simulink model "sensor_fusion"  (R2017b)
settings: Solver=ode45  StartTime=0.0  StopTime=inf  FixedStep=0.1  RelTol=1e-3  EnableMultiTasking=on
PreLoadFcn:
  | RTWConfigurationCB('preloadfcn', bdroot);
InitFcn:
  | parameterVehicle
  | parameterGNC
StopFcn:
  | %myAnimation(xActEst,yActEst,thetaActEst,X_array,Y_array,rp1,rp2)
  | myStopFcn2sim(xEst,yEst,X_array,Y_array,rp1,rp2)
values from neighbouring files (symbols this model uses):
  bDR = 1*b    [parameterGNC.m]
  dcArrayC = [-240 -220 -200 -150 -100 -80 -60 -50 -40 0 40 50    60    80   100   150 200 220 240]    [parameterGNC.m]
  eTickDR = eTick    [parameterGNC.m]
  KP1 = 15    [parameterGNC.m]
  KP2 = 100    [parameterGNC.m]
  rNominalDR = rNominal    [parameterGNC.m]
  rp1 = 0.5    [parameterGNC.m]
  rp2 = 0.2    [parameterGNC.m]
  Tau1 = 0.01    [parameterGNC.m]
  Tau2 = 0.1    [parameterGNC.m]
  TauEncoderDR = 0.01    [parameterGNC.m]
  Tsample = 1/100    (= 0.01)    [parameterGNC.m]
  TsampleEncoderDR = TsampleEncoder    [parameterGNC.m]
  Vcom = 3*VmaxDR/4    [parameterGNC.m]
  wArrayC = [-4.6279   -4.1707   -3.6703   -2.4511   -1.0693   -0.8382   -0.4348   -0.3287 -0.000001 0 0.000001 0.3292    0.4343    0.8065    1.0897    2.3927    3.6855    4.2037    4.6126]./rNominal    [parameterGNC.m]
  X_array = [1 1 0 0]    [parameterGNC.m]
  Y_array = [0 1 1 0]    [parameterGNC.m]
undefined symbols (not defined in the file or in its folder): DiscIntNeverNeededParam
libraries: simulink x17, robotlib x10, aerolibanimutils x1
CloseFcn:
  | rtwprivate ssgencode ModelCloseRequest track_vehicle6_v2
settings Model: Creator=Dogan  LastModifiedBy=uvs4
settings DataIOCC: LimitDataPoints=on  SaveFormat=Array  SignalLoggingSaveFormat=ModelDataLogs
settings OptimizationCC: ExpressionDepthLimit=2147483647  InitFltsAndDblsToZero=on  LifeSpan=inf
settings DebuggingCC: SaveWithParameterizedLinksMsg=none  UnderspecifiedInitializationDetection=Classic  MergeDetectMultiDrivingBlocksExec=none  SignalResolutionControl=TryResolveAllWithWarning  SolverPrmCheckMsg=warning  MultiTaskDSMMsg=warning  MultiTaskCondExecSysMsg=none  FcnCallInpInsideContextMsg=warning  StateNameClashWarn=warning  SFUnexpectedBacktrackingDiag=warning  SFNoUnconditionalDefaultTransitionDiag=warning  SFExecutionAtInitializationDiag=none
settings HardwareCC: ProdBitPerLong=64  ProdLargestAtomicFloat=None  ProdHWDeviceType=Intel->x86-64  TargetHWDeviceType=32-bit Generic
settings ModelReferenceCC: PropagateSignalLabelsOutOfModel=off
settings SFSimCC: SimParseCustomCode=off
settings RTWCC: Description=Generic Real-Time Target
settings CodeAppCC: GenerateComments=off  SimulinkBlockComments=off
settings GRTTargetCC: TargetLangStandard=C89/C90 (ANSI)  GeneratePreprocessorConditionals=Disable all
settings ConfigComp: CovMetricSettings=dw  CovHtmlReporting=on  CovSaveCumulativeToWorkspaceVar=on  CovSaveSingleToWorkspaceVar=on  CovExternalEMLEnable=off

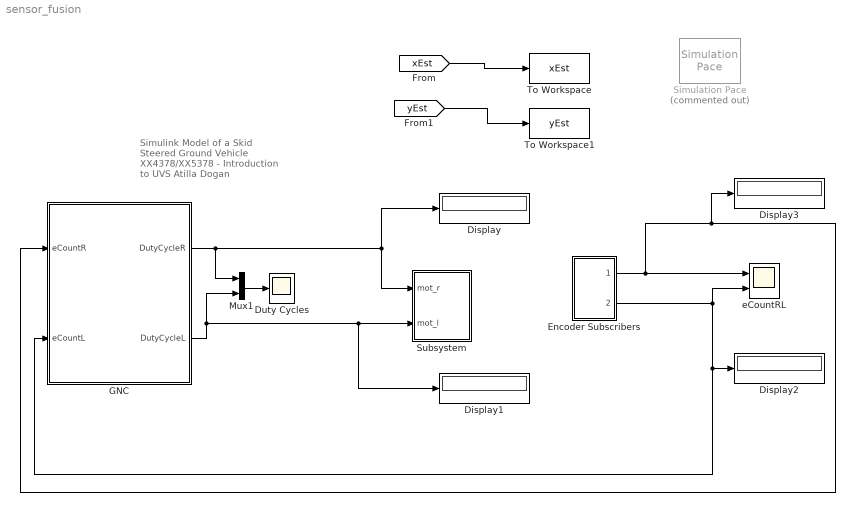
== system sensor_fusion ==
  note: Simulink Model of a Skid Steered Ground Vehicle
      | XX4378/XX5378 - Introduction to UVS
      | Atilla Dogan
  Display{,1..3} (4 alike) : Display
  Duty Cycles : Scope
  Encoder Subscribers : Subsystem
  GNC : Subsystem
  Mux1 : Mux  Inputs=2
  Simulation Pace : aerolibanimutils/Simulation Pace  Commented=on  SimulationPace=1  SleepMode=MATLAB Thread  OutputPaceError=off  SampleTime=1/30
  Subsystem : Subsystem
  To Workspace : ToWorkspace  VariableName=xEst  SaveFormat=Structure With Time  SampleTime=-1
  To Workspace1 : ToWorkspace  VariableName=yEst  SaveFormat=Structure With Time  SampleTime=-1
  eCountRL : Scope  NumInputPorts=2
  wires:
  Mux1/1 -> Duty Cycles/1
  [xEst] -> To Workspace/1
  [yEst] -> To Workspace1/1
  GNC/1(DutyCycleR) -> Mux1/1, Display/1, Subsystem/1(mot_r)
  GNC/2(DutyCycleL) -> Subsystem/2(mot_l), Display1/1, Mux1/2
  Encoder Subscribers/1(enco_R) -> Display3/1, GNC/1(eCountR), eCountRL/1
  Encoder Subscribers/2(enco_L) -> Display2/1, GNC/2(eCountL), eCountRL/2

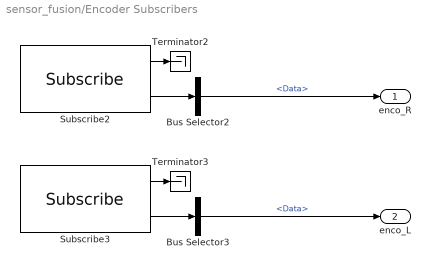
== system sensor_fusion/Encoder Subscribers ==
  Bus Selector2 : BusSelector  OutputSignals=Data
  Bus Selector3 : BusSelector  OutputSignals=Data
  Subscribe2 : robotlib/Subscribe  SourceLibraryInfo=This block requires Robotics System Toolbox  topicSource=Specify your own  topic=/enco_R  messageType=std_msgs/Int16  sampleTime=-1  messageQueueLength=1
      settings: SourceProductBaseCode=RO
  Subscribe3 : robotlib/Subscribe  SourceLibraryInfo=This block requires Robotics System Toolbox  topicSource=Specify your own  topic=/enco_L  messageType=std_msgs/Int16  sampleTime=-1  messageQueueLength=1
      settings: SourceProductBaseCode=RO
  Terminator2 : Terminator
  Terminator3 : Terminator
  enco_R : Outport
  enco_L : Outport  Port=2
  wires:
  Subscribe2/2 -> Bus Selector2/1
  Subscribe2/1 -> Terminator2/1
  Subscribe3/2 -> Bus Selector3/1
  Bus Selector3/1 -> enco_L/1  "<Data>"
  Bus Selector2/1 -> enco_R/1  "<Data>"
  Subscribe3/1 -> Terminator3/1

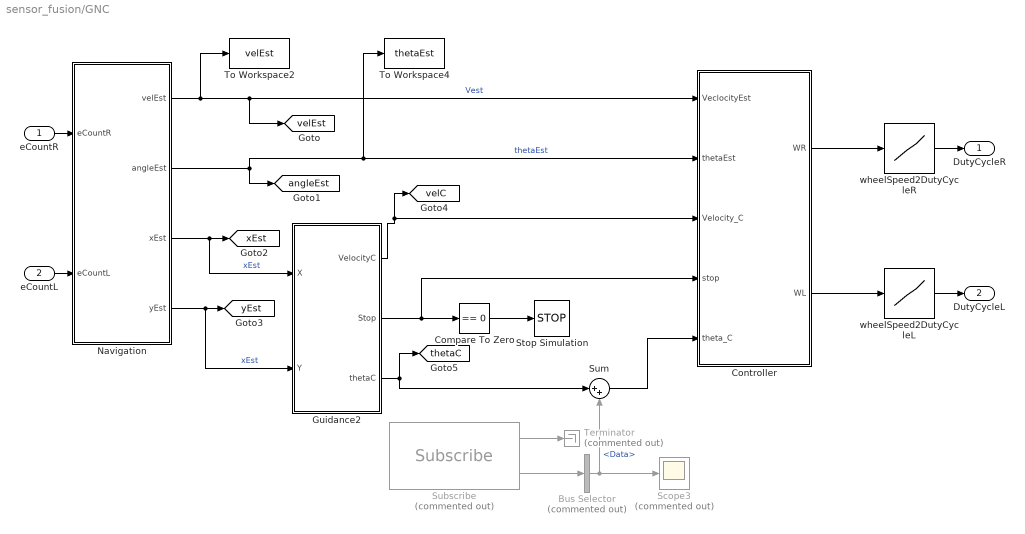
== system sensor_fusion/GNC ==
  eCountR : Inport
  eCountL : Inport  Port=2
  Bus Selector : BusSelector  Commented=on  OutputSignals=Data
  Compare To Zero : simulink/Logic and Bit Operations/Compare To Zero  relop===  OutDataTypeStr=boolean
  Controller : Subsystem
  Guidance2 : Subsystem
  "Navigation " : Subsystem
  Scope3 : Scope  Commented=on
  Stop Simulation : Stop
  Subscribe : robotlib/Subscribe  Commented=on  SourceLibraryInfo=This block requires Robotics System Toolbox  topicSource=Specify your own  topic=/theta_deflection  messageType=std_msgs/Float64  sampleTime=-1  messageQueueLength=1
      settings: SourceProductBaseCode=RO
  Sum : Sum  Inputs=|++
  Terminator : Terminator  Commented=on
  To Workspace2 : ToWorkspace  VariableName=velEst  SampleTime=-1
      settings: Save2DSignal=2-D array (concatenate along first dimension)
  To Workspace4 : ToWorkspace  VariableName=thetaEst  SampleTime=-1
      settings: Save2DSignal=2-D array (concatenate along first dimension)
  wheelSpeed2DutyCycleL : Lookup  InputValues=wArrayC  Table=dcArrayC  LookUpMeth=Interpolation-Use End Values
  wheelSpeed2DutyCycleR : Lookup  InputValues=wArrayC  Table=dcArrayC  LookUpMeth=Interpolation-Use End Values
  DutyCycleR : Outport
  DutyCycleL : Outport  Port=2
  tag scope: angleEst=global, thetaC=global, velC=global, velEst=global, xEst=global, yEst=global
  wires:
  Guidance2/2(Stop) -> Controller/4(stop), Compare To Zero/1
  Controller/1(WR) -> wheelSpeed2DutyCycleR/1
  "Navigation "/4(yEst) -> Guidance2/2(Y), [yEst]  "xEst"
  "Navigation "/3(xEst) -> Guidance2/1(X), [xEst]  "xEst"
  "Navigation "/2(angleEst) -> To Workspace4/1, Controller/2(thetaEst), [angleEst]  "thetaEst"
  "Navigation "/1(velEst) -> To Workspace2/1, Controller/1(VeclocityEst), [velEst]  "Vest"
  eCountL/1 -> "Navigation "/2(eCountL)
  eCountR/1 -> "Navigation "/1(eCountR)
  Guidance2/1(VelocityC) -> Controller/3(Velocity_C), [velC]
  wheelSpeed2DutyCycleR/1 -> DutyCycleR/1
  Controller/2(WL) -> wheelSpeed2DutyCycleL/1
  wheelSpeed2DutyCycleL/1 -> DutyCycleL/1
  Compare To Zero/1 -> Stop Simulation/1
  Guidance2/3(thetaC) -> Sum/1, [thetaC]
  Subscribe/1 -> Terminator/1
  Subscribe/2 -> Bus Selector/1
  Bus Selector/1 -> Sum/2, Scope3/1  "<Data>"
  Sum/1 -> Controller/5(theta_C)

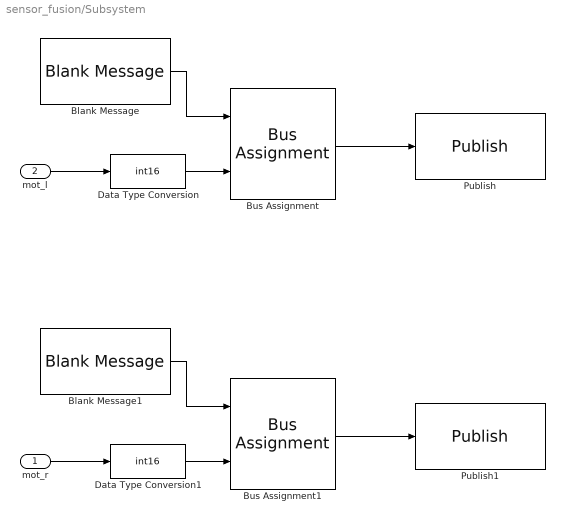
== system sensor_fusion/Subsystem ==
  mot_r : Inport
  mot_l : Inport  Port=2
  Blank Message : robotlib/Blank Message  SourceLibraryInfo=This block requires Robotics System Toolbox  messageType=std_msgs/Int16  SampleTime=inf
      settings: SourceProductBaseCode=RO
  Blank Message1 : robotlib/Blank Message  SourceLibraryInfo=This block requires Robotics System Toolbox  messageType=std_msgs/Int16  SampleTime=inf
      settings: SourceProductBaseCode=RO
  Bus Assignment : BusAssignment  AssignedSignals=Data
  Bus Assignment1 : BusAssignment  AssignedSignals=Data
  Data Type Conversion : DataTypeConversion  OutDataTypeStr=int16
  Data Type Conversion1 : DataTypeConversion  OutDataTypeStr=int16
  Publish : robotlib/Publish  SourceLibraryInfo=This block requires Robotics System Toolbox  topicSource=Specify your own  topic=/pwm_cmd_l  messageType=std_msgs/Int16  messageQueueLength=1
      settings: SourceProductBaseCode=RO
  Publish1 : robotlib/Publish  SourceLibraryInfo=This block requires Robotics System Toolbox  topicSource=Specify your own  topic=/pwm_cmd_r  messageType=std_msgs/Int16  messageQueueLength=1
      settings: SourceProductBaseCode=RO
  wires:
  Bus Assignment/1 -> Publish/1
  Data Type Conversion/1 -> Bus Assignment/2
  Blank Message/1 -> Bus Assignment/1
  mot_l/1 -> Data Type Conversion/1
  mot_r/1 -> Data Type Conversion1/1
  Blank Message1/1 -> Bus Assignment1/1
  Data Type Conversion1/1 -> Bus Assignment1/2
  Bus Assignment1/1 -> Publish1/1

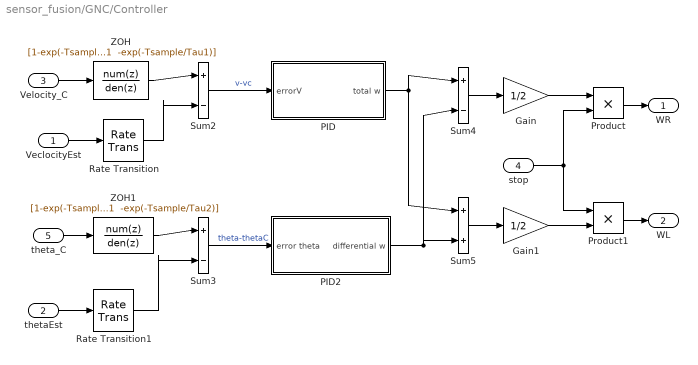
== system sensor_fusion/GNC/Controller ==
  VeclocityEst : Inport
  thetaEst : Inport  Port=2
  Velocity_C : Inport  Port=3
  stop : Inport  Port=4
  theta_C : Inport  Port=5
  Gain : Gain  Gain=1/2
  Gain1 : Gain  Gain=1/2
  PID : Subsystem
  PID2 : Subsystem
  Product : Product  RndMeth=Zero
  Product1 : Product  RndMeth=Zero
  Rate Transition : RateTransition  Deterministic=off
  Rate Transition1 : RateTransition  Deterministic=off
  Sum2 : Sum  Inputs=|+|-|  SampleTime=Tsample
  Sum3 : Sum  Inputs=|+|-|  SampleTime=Tsample
  Sum4 : Sum  Inputs=+|-
  Sum5 : Sum  Inputs=+|+
  ZOH : DiscreteTransferFcn  Numerator=[1-exp(-Tsample/Tau1)]  Denominator="[1  -exp(-Tsample/Tau1)]"  SampleTime=Tsample
  ZOH1 : DiscreteTransferFcn  Numerator=[1-exp(-Tsample/Tau2)]  Denominator="[1  -exp(-Tsample/Tau2)]"  SampleTime=Tsample
  WR : Outport
  WL : Outport  Port=2
  wires:
  Product1/1 -> WL/1
  Product/1 -> WR/1
  Sum5/1 -> Gain1/1
  stop/1 -> Product/2, Product1/1
  Sum4/1 -> Gain/1
  PID2/1(differential w) -> Sum5/2, Sum4/2
  PID/1(total w) -> Sum5/1, Sum4/1
  theta_C/1 -> ZOH1/1
  thetaEst/1 -> Rate Transition1/1
  Velocity_C/1 -> ZOH/1
  VeclocityEst/1 -> Rate Transition/1
  Sum2/1 -> PID/1(errorV)  "v-vc"
  Sum3/1 -> PID2/1(error theta)  "theta-thetaC"
  ZOH/1 -> Sum2/1
  Rate Transition/1 -> Sum2/2
  ZOH1/1 -> Sum3/1
  Rate Transition1/1 -> Sum3/2
  Gain/1 -> Product/1
  Gain1/1 -> Product1/2

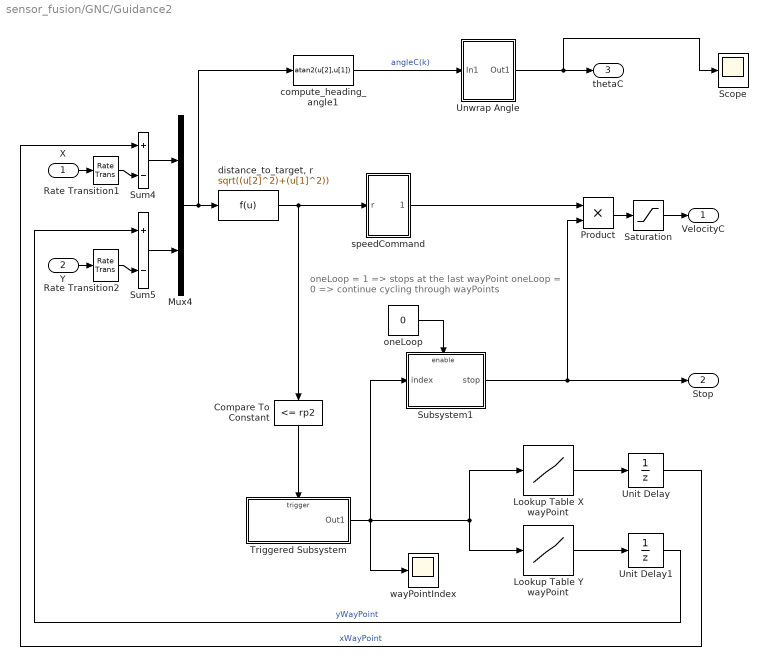
== system sensor_fusion/GNC/Guidance2 ==
  note: oneLoop = 1 => stops at the last wayPoint
      | oneLoop = 0 => continue cycling through wayPoints
  X : Inport
  Y : Inport  Port=2
  Compare To Constant : simulink/Logic and Bit Operations/Compare To Constant  relop=<=  const=rp2  OutDataTypeStr=uint8  ZeroCross=off
  Lookup Table X wayPoint : Lookup  InputValues=[1:length(X_array)]  Table=X_array  LookUpMeth=Interpolation-Use End Values  OutDataTypeStr=double
  Lookup Table Y wayPoint : Lookup  InputValues=[1:length(Y_array)]  Table=Y_array  LookUpMeth=Interpolation-Use End Values  OutDataTypeStr=double
  Mux4 : Mux  Inputs=2
  Product : Product  RndMeth=Zero
  Rate Transition1 : RateTransition
  Rate Transition2 : RateTransition
  Saturation : Saturate  UpperLimit=Vcom  LowerLimit=0  SampleTime=Tsample
  Scope : Scope
  Subsystem1 : Subsystem
  Sum4 : Sum  Inputs=|+|-|
  Sum5 : Sum  Inputs=|+|-|
  Triggered Subsystem : Subsystem  TreatAsAtomicUnit=on
  Unit Delay : UnitDelay  SampleTime=Tsample
  Unit Delay1 : UnitDelay  SampleTime=Tsample
  Unwrap Angle : Subsystem
  compute_heading_angle1 : Fcn  Expr=atan2(u[2],u[1])  SampleTime=Tsample
  "distance_to_target, r" : Fcn  Expr=sqrt((u[2]^2)+(u[1]^2))  SampleTime=Tsample
  oneLoop : Constant  Value=0  OutDataTypeStr=uint32  SampleTime=Tsample
  speedCommand : Subsystem
  wayPointIndex : Scope
  VelocityC : Outport
  Stop : Outport  Port=2
  thetaC : Outport  Port=3
  wires:
  speedCommand/1(Vdes) -> Product/1
  Sum4/1 -> Mux4/1
  "distance_to_target, r"/1 -> Compare To Constant/1, speedCommand/1(r)
  Lookup Table X wayPoint/1 -> Unit Delay/1
  Lookup Table Y wayPoint/1 -> Unit Delay1/1
  X/1 -> Rate Transition1/1
  Y/1 -> Rate Transition2/1
  Sum5/1 -> Mux4/2
  Compare To Constant/1 -> Triggered Subsystem/Trigger
  Triggered Subsystem/1(Out1) -> Subsystem1/1(index), wayPointIndex/1, Lookup Table X wayPoint/1, Lookup Table Y wayPoint/1
  Unit Delay/1 -> Sum4/1  "xWayPoint"
  Unit Delay1/1 -> Sum5/1  "yWayPoint"
  Saturation/1 -> VelocityC/1
  Rate Transition1/1 -> Sum4/2
  Rate Transition2/1 -> Sum5/2
  Product/1 -> Saturation/1
  Subsystem1/1(stop) -> Product/2, Stop/1
  oneLoop/1 -> Subsystem1/Enable
  Mux4/1 -> compute_heading_angle1/1, "distance_to_target, r"/1
  compute_heading_angle1/1 -> Unwrap Angle/1(In1)  "angleC(k)"
  Unwrap Angle/1(Out1) -> thetaC/1, Scope/1

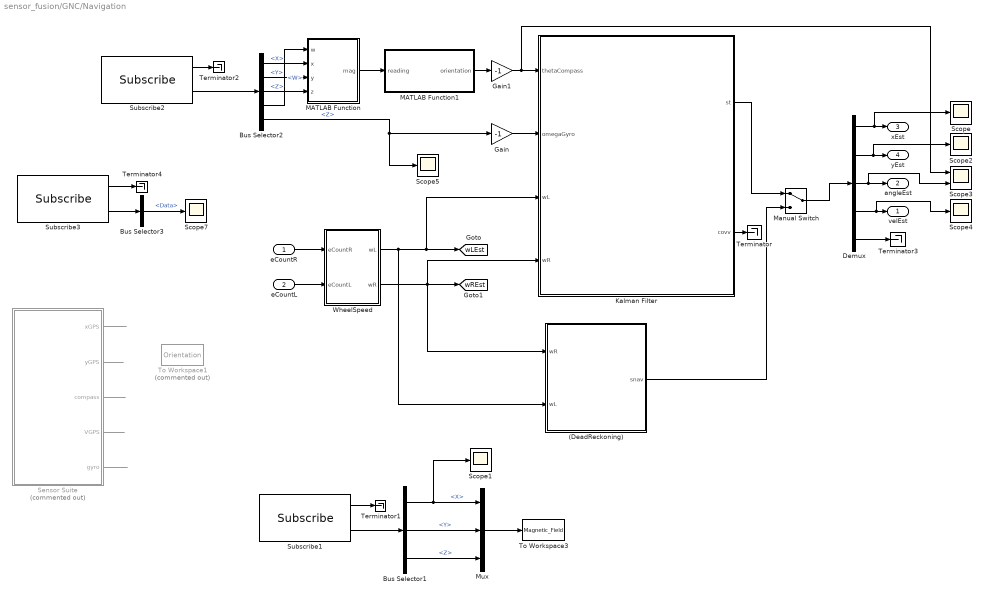
== system sensor_fusion/GNC/Navigation  ==
  eCountR : Inport
  eCountL : Inport  Port=2
  (DeadReckoning) : Subsystem
  Bus Selector1 : BusSelector  OutputSignals=MagneticField_.X,MagneticField_.Y,MagneticField_.Z
  Bus Selector2 : BusSelector  OutputSignals=Orientation.X,Orientation.Y,Orientation.Z,Orientation.W,AngularVelocity.Z
  Bus Selector3 : BusSelector  OutputSignals=Data
  Demux : Demux  Outputs=5
  Gain : Gain  Gain=-1
  Gain1 : Gain  Gain=-1
  Kalman Filter : MATLAB Function  TreatAsAtomicUnit=on  SystemSampleTime=Tsample
  MATLAB Function : MATLAB Function  TreatAsAtomicUnit=on
  MATLAB Function1 : MATLAB Function  TreatAsAtomicUnit=on
  Manual Switch : ManualSwitch
  Mux : Mux  Inputs=3
  Scope{,1..2,4..5,7} (6 alike) : Scope
  Scope3 : Scope  NumInputPorts=2
  Sensor Suite : Subsystem  Commented=on
  Subscribe1 : robotlib/Subscribe  SourceLibraryInfo=This block requires Robotics System Toolbox  topicSource=Specify your own  topic=/mavros/imu/mag  messageType=sensor_msgs/MagneticField  sampleTime=Tsample  messageQueueLength=1
      settings: SourceProductBaseCode=RO
  Subscribe2 : robotlib/Subscribe  SourceLibraryInfo=This block requires Robotics System Toolbox  topicSource=Specify your own  topic=/mavros/imu/data  messageType=sensor_msgs/Imu  sampleTime=Tsample  messageQueueLength=1
      settings: SourceProductBaseCode=RO
  Subscribe3 : robotlib/Subscribe  SourceLibraryInfo=This block requires Robotics System Toolbox  topicSource=Specify your own  topic=/mavros/global_position/compass_hdg  messageType=std_msgs/Float64  sampleTime=Tsample  messageQueueLength=1
      settings: SourceProductBaseCode=RO
  Terminator{,1..4} (5 alike) : Terminator
  To Workspace1 : ToWorkspace  Commented=on  VariableName=Orientation  SampleTime=-1
      settings: Save2DSignal=2-D array (concatenate along first dimension)
  To Workspace3 : ToWorkspace  VariableName=Magnetic_Field  SampleTime=-1
      settings: Save2DSignal=2-D array (concatenate along first dimension)
  WheelSpeed : Subsystem
  velEst : Outport
  angleEst : Outport  Port=2
  xEst : Outport  Port=3
  yEst : Outport  Port=4
  tag scope: wLEst=global, wREst=global
  wires:
  WheelSpeed/2(wR) -> (DeadReckoning)/1(wR), Kalman Filter/4(wR), [wREst]
  eCountL/1 -> WheelSpeed/2(eCountL)
  eCountR/1 -> WheelSpeed/1(eCountR)
  Sensor Suite/1(xGPS) -> ?
  Sensor Suite/2(yGPS) -> ?
  Sensor Suite/3(compass) -> ?
  Sensor Suite/4(VGPS) -> ?
  Sensor Suite/5(gyro) -> ?
  Demux/1 -> Scope/1, xEst/1
  Demux/2 -> Scope2/1, yEst/1
  Demux/3 -> Scope3/2, angleEst/1
  Demux/4 -> Scope4/1, velEst/1
  Kalman Filter/1(st) -> Manual Switch/1
  (DeadReckoning)/1(snav) -> Manual Switch/2
  Manual Switch/1 -> Demux/1
  WheelSpeed/1(wL) -> (DeadReckoning)/2(wL), Kalman Filter/3(wL), [wLEst]
  Mux/1 -> To Workspace3/1
  Bus Selector1/2 -> Mux/2  "<Y>"
  Bus Selector1/3 -> Mux/3  "<Z>"
  Bus Selector1/1 -> Mux/1, Scope1/1  "<X>"
  Subscribe2/2 -> Bus Selector2/1
  Subscribe2/1 -> Terminator2/1
  Subscribe1/1 -> Terminator1/1
  Subscribe1/2 -> Bus Selector1/1
  Bus Selector2/1 -> MATLAB Function/2(x)  "<X>"
  Bus Selector2/2 -> MATLAB Function/3(y)  "<Y>"
  Bus Selector2/3 -> MATLAB Function/4(z)  "<Z>"
  Bus Selector2/4 -> MATLAB Function/1(w)  "<W>"
  Bus Selector2/5 -> Gain/1, Scope5/1  "<Z>"
  Kalman Filter/2(covv) -> Terminator/1
  Demux/5 -> Terminator3/1
  Subscribe3/2 -> Bus Selector3/1
  Subscribe3/1 -> Terminator4/1
  Bus Selector3/1 -> Scope7/1  "<Data>"
  MATLAB Function/1(mag) -> MATLAB Function1/1(reading)
  MATLAB Function1/1(orientation) -> Gain1/1
  Gain/1 -> Kalman Filter/2(omegaGyro)
  Gain1/1 -> Kalman Filter/1(thetaCompass), Scope3/1

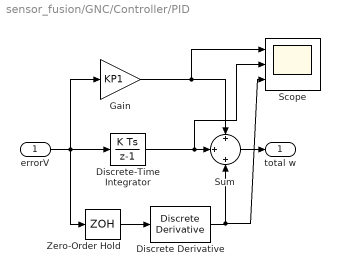
== system sensor_fusion/GNC/Controller/PID ==
  errorV : Inport
  Discrete Derivative : simulink/Discrete/Discrete Derivative  gainval=KD1  ICPrevScaledInput=0.0  InputProcessing=Inherited  OutMin=[]  OutMax=[]  OutDataType=sfix(16)  OutScaling=2^-10  DoSatur=off
  Discrete-Time Integrator : DiscreteIntegrator  gainval=KI1  SampleTime=Tsample  ICPrevOutput=DiscIntNeverNeededParam  ICPrevScaledInput=DiscIntNeverNeededParam
  Gain : Gain  Gain=KP1  SampleTime=Tsample
  Scope : Scope  NumInputPorts=3
  Sum : Sum  Inputs=+|+|+
  Zero-Order Hold : ZeroOrderHold  SampleTime=Tsample
  total w : Outport
  wires:
  Discrete Derivative/1 -> Scope/3, Sum/3
  Zero-Order Hold/1 -> Discrete Derivative/1
  Gain/1 -> Scope/1, Sum/1
  errorV/1 -> Discrete-Time Integrator/1, Gain/1, Zero-Order Hold/1
  Sum/1 -> total w/1
  Discrete-Time Integrator/1 -> Scope/2, Sum/2

== system sensor_fusion/GNC/Controller/PID2 ==
  error theta : Inport
  Discrete Derivative1 : simulink/Discrete/Discrete Derivative  gainval=KD2  ICPrevScaledInput=0.0  InputProcessing=Inherited  OutMin=[]  OutMax=[]  OutDataType=sfix(16)  OutScaling=2^-10  DoSatur=off
  Discrete-Time Integrator1 : DiscreteIntegrator  gainval=KI2  SampleTime=Tsample  ICPrevOutput=DiscIntNeverNeededParam  ICPrevScaledInput=DiscIntNeverNeededParam
  Gain1 : Gain  Gain=KP2  SampleTime=Tsample
  Scope1 : Scope  NumInputPorts=3
  Sum1 : Sum  Inputs=+|+|+
  Zero-Order Hold1 : ZeroOrderHold  SampleTime=Tsample
  differential w : Outport
  wires:
  Discrete Derivative1/1 -> Scope1/3, Sum1/3
  Zero-Order Hold1/1 -> Discrete Derivative1/1
  error theta/1 -> Gain1/1, Discrete-Time Integrator1/1, Zero-Order Hold1/1
  Discrete-Time Integrator1/1 -> Scope1/2, Sum1/2
  Gain1/1 -> Scope1/1, Sum1/1
  Sum1/1 -> differential w/1

== system sensor_fusion/GNC/Guidance2/Subsystem1 ==
  note: NAND = TRUE
      | if at least one input is FALSE
      |
      | NAND = FALSE
      | if both inputs are TRUE
  index : Inport
  Enable : EnablePort
  Compare To Constant1 : simulink/Logic and Bit Operations/Compare To Constant  relop===  const=1  OutDataTypeStr=uint8  ZeroCross=off
  Compare To Constant2 : simulink/Logic and Bit Operations/Compare To Constant  relop===  const=length(X_array)  OutDataTypeStr=uint8  ZeroCross=off
  Logical Operator1 : Logic  Operator=NAND  IconShape=distinctive  AllPortsSameDT=off  OutDataTypeStr=boolean
  Triggered Subsystem2 : Subsystem  TreatAsAtomicUnit=on
  stop : Outport  OutputWhenDisabled=reset  InitialOutput=[1]
  wires:
  Logical Operator1/1 -> stop/1
  index/1 -> Compare To Constant1/1, Compare To Constant2/1
  Compare To Constant1/1 -> Logical Operator1/1
  Triggered Subsystem2/1(Out1) -> Logical Operator1/2
  Compare To Constant2/1 -> Triggered Subsystem2/Trigger

== system sensor_fusion/GNC/Guidance2/Triggered Subsystem ==
  Trigger : TriggerPort  VariantControl=Variant
  Compare To Constant1 : simulink/Logic and Bit Operations/Compare To Constant  relop=>=  const=length(X_array)  OutDataTypeStr=uint8  ZeroCross=off
  CountReset : Constant  OutDataTypeStr=uint32  SampleTime=-1
  Sum3 : Sum  OutDataTypeStr=uint32
  Switch : Switch  Threshold=0.5
  Unit Delay : UnitDelay  InitialCondition=1  SampleTime=-1
  countIncrement : Constant  OutDataTypeStr=uint32  SampleTime=-1
  Out1 : Outport  OutDataTypeStr=uint32  InitialOutput=1
  wires:
  countIncrement/1 -> Sum3/2
  Unit Delay/1 -> Compare To Constant1/1, Sum3/1
  Compare To Constant1/1 -> Switch/2
  Switch/1 -> Out1/1, Unit Delay/1
  CountReset/1 -> Switch/1
  Sum3/1 -> Switch/3

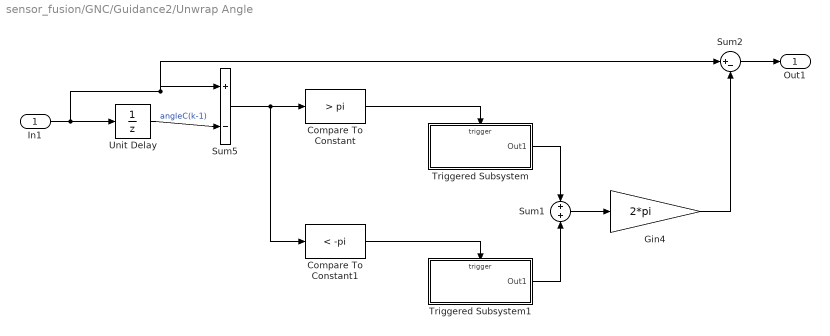
== system sensor_fusion/GNC/Guidance2/Unwrap Angle ==
  In1 : Inport
  Compare To Constant : simulink/Logic and Bit Operations/Compare To Constant  relop=>  const=pi  OutDataTypeStr=uint8  ZeroCross=off
  Compare To Constant1 : simulink/Logic and Bit Operations/Compare To Constant  relop=<  const=-pi  OutDataTypeStr=uint8  ZeroCross=off
  Gin4 : Gain  Gain=2*pi  OutDataTypeStr=double  SampleTime=Tsample
  Sum1 : Sum  Inputs=+|+
  Sum2 : Sum  Inputs=|+-
  Sum5 : Sum  Inputs=|+|-|
  Triggered Subsystem : Subsystem  TreatAsAtomicUnit=on
  Triggered Subsystem1 : Subsystem  TreatAsAtomicUnit=on
  Unit Delay : UnitDelay  SampleTime=Tsample
  Out1 : Outport
  wires:
  In1/1 -> Unit Delay/1, Sum5/1, Sum2/1
  Unit Delay/1 -> Sum5/2  "angleC(k-1)"
  Sum5/1 -> Compare To Constant/1, Compare To Constant1/1
  Compare To Constant1/1 -> Triggered Subsystem1/Trigger
  Compare To Constant/1 -> Triggered Subsystem/Trigger
  Triggered Subsystem/1(Out1) -> Sum1/1
  Triggered Subsystem1/1(Out1) -> Sum1/2
  Sum1/1 -> Gin4/1
  Sum2/1 -> Out1/1
  Gin4/1 -> Sum2/2

== system sensor_fusion/GNC/Guidance2/speedCommand ==
  r : Inport
  Compare To Constant2 : simulink/Logic and Bit Operations/Compare To Constant  relop=>  const=rp1  OutDataTypeStr=uint8  ZeroCross=off
  Gin4 : Gain  Gain=0.1  SampleTime=Tsample
  Manual Switch : ManualSwitch  CurrentSetting=0
  Switch : Switch  Criteria=u2 > Threshold
  Vcom : Constant  Value=Vcom  SampleTime=Tsample
  Vcom1 : Constant  Value=Vcom  SampleTime=Tsample
  Vdes : Outport
  wires:
  Compare To Constant2/1 -> Switch/2
  Vcom/1 -> Switch/1
  Vcom1/1 -> Manual Switch/2
  Switch/1 -> Manual Switch/1
  Gin4/1 -> Switch/3
  r/1 -> Compare To Constant2/1, Gin4/1
  Manual Switch/1 -> Vdes/1

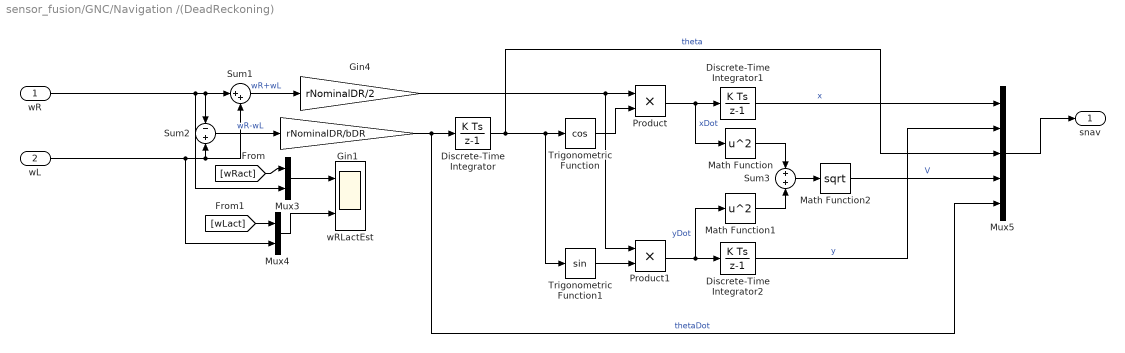
== system sensor_fusion/GNC/Navigation /(DeadReckoning) ==
  wR : Inport
  wL : Inport  Port=2
  Discrete-Time Integrator : DiscreteIntegrator  SampleTime=TsampleEncoderDR  ICPrevOutput=DiscIntNeverNeededParam  ICPrevScaledInput=DiscIntNeverNeededParam
  Discrete-Time Integrator1 : DiscreteIntegrator  SampleTime=TsampleEncoderDR  ICPrevOutput=DiscIntNeverNeededParam  ICPrevScaledInput=DiscIntNeverNeededParam
  Discrete-Time Integrator2 : DiscreteIntegrator  SampleTime=TsampleEncoderDR  ICPrevOutput=DiscIntNeverNeededParam  ICPrevScaledInput=DiscIntNeverNeededParam
  Gin1 : Gain  Gain=rNominalDR/bDR  OutDataTypeStr=double
  Gin4 : Gain  Gain=rNominalDR/2  OutDataTypeStr=double
  Math Function : Math  Operator=square  SaturateOnIntegerOverflow=on
  Math Function1 : Math  Operator=square  SaturateOnIntegerOverflow=on
  Math Function2 : Math  Operator=sqrt  OutputSignalType=real  SaturateOnIntegerOverflow=on
  Mux3 : Mux  Inputs=2
  Mux4 : Mux  Inputs=2
  Mux5 : Mux  Inputs=5
  Product : Product  RndMeth=Zero
  Product1 : Product  RndMeth=Zero
  Sum1 : Sum  Inputs=|++
  Sum2 : Sum  Inputs=-|+
  Sum3 : Sum  Inputs=+|+
  Trigonometric Function : Trigonometry  Operator=cos  OutputSignalType=real
  Trigonometric Function1 : Trigonometry  OutputSignalType=real
  wRLactEst : Scope  NumInputPorts=2
  snav : Outport
  wires:
  [wLact] -> Mux4/1
  [wRact] -> Mux3/1
  Mux4/1 -> wRLactEst/2
  Mux3/1 -> wRLactEst/1
  Math Function2/1 -> Mux5/4  "V"
  Sum3/1 -> Math Function2/1
  Math Function1/1 -> Sum3/2
  Math Function/1 -> Sum3/1
  Discrete-Time Integrator2/1 -> Mux5/2  "y"
  Discrete-Time Integrator1/1 -> Mux5/1  "x"
  Product1/1 -> Math Function1/1, Discrete-Time Integrator2/1  "yDot"
  Product/1 -> Math Function/1, Discrete-Time Integrator1/1  "xDot"
  Trigonometric Function1/1 -> Product1/2
  Gin4/1 -> Product1/1, Product/1
  Trigonometric Function/1 -> Product/2
  Discrete-Time Integrator/1 -> Mux5/3, Trigonometric Function1/1, Trigonometric Function/1  "theta"
  Gin1/1 -> Mux5/5, Discrete-Time Integrator/1  "thetaDot"
  Sum2/1 -> Gin1/1  "wR-wL"
  Sum1/1 -> Gin4/1  "wR+wL"
  wR/1 -> Mux3/2, Sum2/1, Sum1/1
  wL/1 -> Mux4/2, Sum2/2, Sum1/2
  Mux5/1 -> snav/1

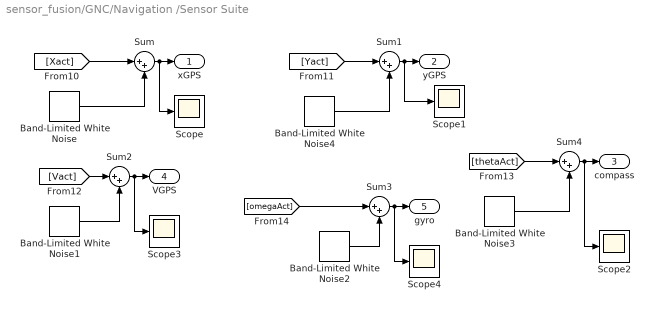
== system sensor_fusion/GNC/Navigation /Sensor Suite ==
  Band-Limited White Noise : simulink/Sources/Band-Limited White Noise  Cov=[0.01]  Ts=0.1  seed=[23341]
  Band-Limited White Noise1 : simulink/Sources/Band-Limited White Noise  Cov=[0.1]  Ts=0.1  seed=[23341]
  Band-Limited White Noise2 : simulink/Sources/Band-Limited White Noise  Cov=[0.1]  Ts=0.1  seed=[23341]
  Band-Limited White Noise3 : simulink/Sources/Band-Limited White Noise  Cov=[0.1]  Ts=0.1  seed=[23341]
  Band-Limited White Noise4 : simulink/Sources/Band-Limited White Noise  Cov=[0.01]  Ts=0.1  seed=[23341]
  Scope{,1..4} (5 alike) : Scope
  Sum{,1..4} (5 alike) : Sum  Inputs=|++
  xGPS : Outport
  yGPS : Outport  Port=2
  compass : Outport  Port=3
  VGPS : Outport  Port=4
  gyro : Outport  Port=5
  wires:
  Band-Limited White Noise/1 -> Sum/2
  [omegaAct] -> Sum3/1
  [Yact] -> Sum1/1
  Band-Limited White Noise4/1 -> Sum1/2
  [Vact] -> Sum2/1
  [thetaAct] -> Sum4/1
  [Xact] -> Sum/1
  Band-Limited White Noise2/1 -> Sum3/2
  Band-Limited White Noise3/1 -> Sum4/2
  Band-Limited White Noise1/1 -> Sum2/2
  Sum/1 -> Scope/1, xGPS/1
  Sum1/1 -> Scope1/1, yGPS/1
  Sum2/1 -> Scope3/1, VGPS/1
  Sum4/1 -> Scope2/1, compass/1
  Sum3/1 -> Scope4/1, gyro/1

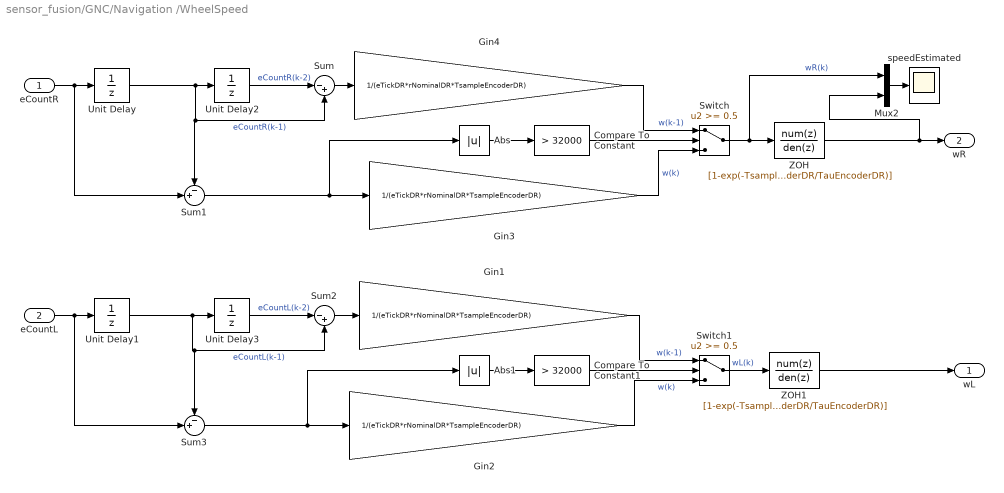
== system sensor_fusion/GNC/Navigation /WheelSpeed ==
  eCountR : Inport
  eCountL : Inport  Port=2
  Abs : Abs
  Abs1 : Abs
  Compare To Constant : simulink/Logic and Bit Operations/Compare To Constant  relop=>  const=32000  OutDataTypeStr=uint8  ZeroCross=off
  Compare To Constant1 : simulink/Logic and Bit Operations/Compare To Constant  relop=>  const=32000  OutDataTypeStr=uint8  ZeroCross=off
  Gin{1..4} (4 alike) : Gain  Gain=1/(eTickDR*rNominalDR*TsampleEncoderDR)  OutDataTypeStr=double  SampleTime=TsampleEncoderDR
  Mux2 : Mux  Inputs=2
  Sum : Sum  Inputs=|-+
  Sum1 : Sum  Inputs=-+|
  Sum2 : Sum  Inputs=|-+
  Sum3 : Sum  Inputs=-+|
  Switch : Switch  Threshold=0.5
  Switch1 : Switch  Threshold=0.5
  Unit Delay{,1..3} (4 alike) : UnitDelay  SampleTime=TsampleEncoderDR
  ZOH : DiscreteTransferFcn  Numerator=[1-exp(-TsampleEncoderDR/TauEncoderDR)]  Denominator="[1  -exp(-TsampleEncoderDR/TauEncoderDR)]"  SampleTime=TsampleEncoderDR
  ZOH1 : DiscreteTransferFcn  Numerator=[1-exp(-TsampleEncoderDR/TauEncoderDR)]  Denominator="[1  -exp(-TsampleEncoderDR/TauEncoderDR)]"  SampleTime=TsampleEncoderDR
  speedEstimated : Scope
  wL : Outport
  wR : Outport  Port=2
  wires:
  Mux2/1 -> speedEstimated/1
  ZOH1/1 -> wL/1
  ZOH/1 -> wR/1, Mux2/2
  Switch1/1 -> ZOH1/1  "wL(k)"
  Switch/1 -> Mux2/1, ZOH/1  "wR(k)"
  Compare To Constant1/1 -> Switch1/2
  Abs1/1 -> Compare To Constant1/1
  Gin2/1 -> Switch1/3  "w(k)"
  Gin1/1 -> Switch1/1  "w(k-1)"
  Sum3/1 -> Gin2/1, Abs1/1
  Sum2/1 -> Gin1/1
  Unit Delay3/1 -> Sum2/1  "eCountL(k-2)"
  Unit Delay1/1 -> Unit Delay3/1, Sum2/2, Sum3/1  "eCountL(k-1)"
  eCountL/1 -> Unit Delay1/1, Sum3/2
  Compare To Constant/1 -> Switch/2
  Abs/1 -> Compare To Constant/1
  Gin3/1 -> Switch/3  "w(k)"
  Gin4/1 -> Switch/1  "w(k-1)"
  Sum1/1 -> Gin3/1, Abs/1
  Sum/1 -> Gin4/1
  Unit Delay2/1 -> Sum/1  "eCountR(k-2)"
  Unit Delay/1 -> Sum1/1, Sum/2, Unit Delay2/1  "eCountR(k-1)"
  eCountR/1 -> Sum1/2, Unit Delay/1

== system sensor_fusion/GNC/Guidance2/Subsystem1/Triggered Subsystem2 ==
  Trigger : TriggerPort  VariantControl=Variant
  Constant : Constant  OutDataTypeStr=uint32  SampleTime=-1
  Out1 : Outport  OutDataTypeStr=uint32  InitialOutput=0
  wires:
  Constant/1 -> Out1/1

== system sensor_fusion/GNC/Guidance2/Unwrap Angle/Triggered Subsystem ==
  Trigger : TriggerPort  VariantControl=Variant
  Sum3 : Sum  OutDataTypeStr=int32
  Unit Delay : UnitDelay  SampleTime=-1
  countIncrement : Constant  OutDataTypeStr=int32  SampleTime=-1
  Out1 : Outport  OutDataTypeStr=int32  InitialOutput=0
  wires:
  countIncrement/1 -> Sum3/2
  Unit Delay/1 -> Sum3/1
  Sum3/1 -> Out1/1, Unit Delay/1

== system sensor_fusion/GNC/Guidance2/Unwrap Angle/Triggered Subsystem1 ==
  Trigger : TriggerPort  VariantControl=Variant
  Sum3 : Sum  Inputs=+-  OutDataTypeStr=int32
  Unit Delay : UnitDelay  SampleTime=-1
  countIncrement : Constant  OutDataTypeStr=int32  SampleTime=-1
  Out1 : Outport  OutDataTypeStr=int32  InitialOutput=0
  wires:
  Sum3/1 -> Out1/1, Unit Delay/1
  Unit Delay/1 -> Sum3/1
  countIncrement/1 -> Sum3/2

== matlab function sensor_fusion/GNC/Navigation /MATLAB Function ==
  data: w input; mag output; x input; y input; z input
function mag = fcn(w,x,y,z)
    eul = quat2eul([w,x,y,z]);
    mag = eul(1);
end

== matlab function sensor_fusion/GNC/Navigation /Kalman Filter ==
  data: thetaCompass input; omegaGyro input; wL input; wR input; st output; Tsample parameter; rNominalDR parameter; bDR parameter; covv output
function [st,covv] =  ExtKalman(thetaCompass,omegaGyro,wL,wR,Tsample,rNominalDR,bDR)
%#codegen
% if thetaCompass<0
%     thetaCompass = 2*pi-thetaCompass;
% end

meas=[thetaCompass;omegaGyro];
%meas=[thetaCompass];
persistent P xhat 
if isempty(P)
   % First time through the code so do some initialization
   xhat = zeros(5,1);
   P = zeros(5,5);
 end 
   Q = diag([0.1 0.1 0.1 1 1]);
  R = 150*diag([1 1]);
%    R = 150;
% Calculate the Jacobians for the state and measurement equations
F = [1 0  -Tsample*xhat(4)*sin(xhat(3)) Tsample*cos(xhat(3)) 0 ;
     0 1   Tsample*xhat(4)*cos(xhat(3)) Tsample*sin(xhat(3)) 0 ;
     0 0            1                 0           Tsample ;
     0 0            0                 0            0 ;
     0 0            0                 0            0 ];
H =[0 0 1 0 0; 0 0 0 0 1];
%H =[0 0 1 0 0];
% Propogate  the state and covariance matrices
xhat = [...
    xhat(1) + Tsample*xhat(4)*cos(xhat(3));
    xhat(2) + Tsample*xhat(4)*sin(xhat(3));
    xhat(3)  + Tsample * xhat(5);
    rNominalDR*(wL+wR)/2;
    rNominalDR*(wL-wR)/bDR];

% if (xhat(3) < -pi) || (pi < xhat(3))    
%     xhat(3) = (xhat(3) + pi);
%     if (xhat(3) > 0)
%     xhat(3) = mod(xhat(3), 2*pi);
%         if(xhat(3) == 0) 
%         xhat(3)= 2*pi;
%         end
%     end
%     xhat(3)=xhat(3) - pi;
% end

P = F*P*F' + Q;
% Calculate the Kalman gain
K = P*H'/(H*P*H' + R);
% Calculate the measurement residual
yhat = H*xhat;
resid = meas - yhat;
% Update the state and covariance estimates
xhat = xhat + K*resid;
P = (eye(size(K,1))-K*H)*P;
% Post the results
st = xhat;
covv = P;

== matlab function sensor_fusion/GNC/Navigation /MATLAB Function1 ==
  data: orientation output; reading input
function orientation = fcn(reading)
    % base all angles relative to the initial one
    persistent first_reading;
    if isempty(first_reading)
        first_reading = reading;
    end
    reading = reading - first_reading;
    
    persistent previous_orientation;
    if isempty(previous_orientation)
        previous_orientation = 0;
    end
    
    c = round((previous_orientation - reading) / (2 * pi));
    orientation = 2 * pi * c + reading;
    
    previous_orientation = orientation;
end
